simulink model "auv_full_system"  (R2026a)
settings: Solver=FixedStepDiscrete  StopTime=90  FixedStep=0.2
settings Model: Creator=muthuraam  LastModifiedBy=muthuraam

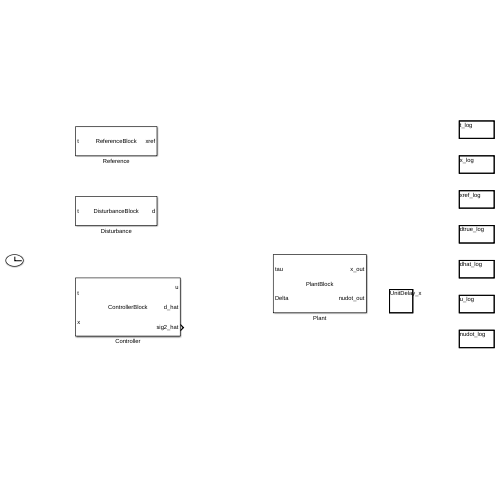
[thumbnail: Simulink's stored preview of the top-level diagram]
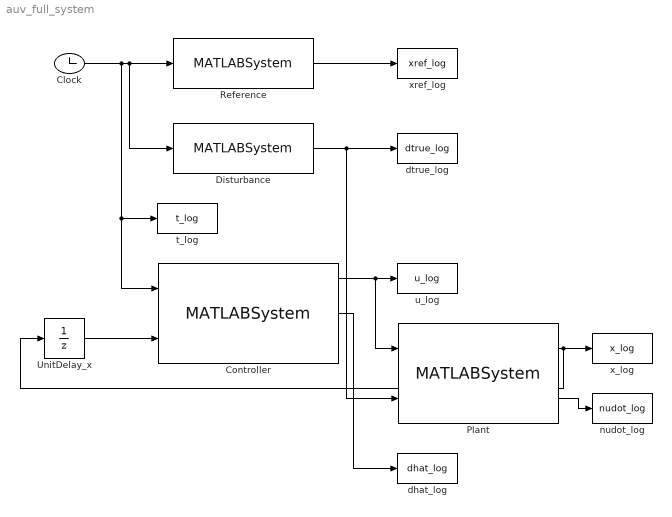
== system auv_full_system ==
  Clock : Clock
  Controller : MATLABSystem  System=ControllerBlock  SimulateUsing=Interpreted execution
      mask Type: ControllerBlock
  Disturbance : MATLABSystem  System=DisturbanceBlock  SimulateUsing=Interpreted execution
      mask Type: DisturbanceBlock
  Plant : MATLABSystem  System=PlantBlock  SimulateUsing=Interpreted execution
      mask Type: PlantBlock
  Reference : MATLABSystem  System=ReferenceBlock  SimulateUsing=Interpreted execution
      mask Type: ReferenceBlock
  UnitDelay_x : UnitDelay  SampleTime=-1
  dhat_log : ToWorkspace  VariableName=dhat_log  SampleTime=-1
  dtrue_log : ToWorkspace  VariableName=dtrue_log  SampleTime=-1
  nudot_log : ToWorkspace  VariableName=nudot_log  SampleTime=-1
  t_log : ToWorkspace  VariableName=t_log  SampleTime=-1
  u_log : ToWorkspace  VariableName=u_log  SampleTime=-1
  x_log : ToWorkspace  VariableName=x_log  SampleTime=-1
  xref_log : ToWorkspace  VariableName=xref_log  SampleTime=-1
  wires:
  Plant/1 -> x_log/1, UnitDelay_x/1
  Controller/1 -> u_log/1, Plant/1
  Reference/1 -> xref_log/1
  Plant/2 -> nudot_log/1
  Disturbance/1 -> dtrue_log/1, Plant/2
  UnitDelay_x/1 -> Controller/2
  Controller/2 -> dhat_log/1
  Clock/1 -> t_log/1, Controller/1, Disturbance/1, Reference/1
